simulink model "r2016bSingleARDroneCtrl"  (R2016b)
settings: Solver=FixedStepAuto  StartTime=0.0  StopTime=inf  FixedStep=sampleTime  RelTol=1e-3  EnableMultiTasking=on
values from neighbouring files (symbols this model uses):
  k_d_xy = 0.5    [start.m]
  k_d_z = 0.3    [start.m]
  k_i_xy = 0.01    [start.m]
  k_p_xy = 0.7    [start.m]
  k_p_yaw = 0.5    [start.m]
  k_p_z = 0.6    [start.m]
  limit_cmd_xy = 10    [start.m]
  waypoints1 = getWaypoints(0)    [start.m]
  waypoints2 = getWaypoints(-pi)    [start.m]
undefined symbols (not defined in the file or in its folder): Angular, Linear
libraries: robotlib x6
settings Model: Creator=exbot  LastModifiedBy=zhenglong
settings DataIOCC: LimitDataPoints=on
settings OptimizationCC: MaxStackSize=64
settings DebuggingCC: ParameterTunabilityLossMsg=error  AllowSymbolicDim=off  SFUnexpectedBacktrackingDiag=warning  SFNoUnconditionalDefaultTransitionDiag=warning  SFExecutionAtInitializationDiag=none
settings HardwareCC: ProdBitPerPointer=32  ProdBitPerSizeT=32  ProdBitPerPtrDiffT=32  ProdLargestAtomicFloat=None  ProdIntDivRoundTo=Undefined  ProdEndianess=Unspecified  ProdWordSize=32  ProdHWDeviceType=Generic->Unspecified (assume 32-bit Generic)
settings ModelReferenceCC: PropagateSignalLabelsOutOfModel=off
settings RTWCC: SystemTargetFile=ert.tlc  HardwareBoard=Robot Operating System (ROS)  TLCOptions="-aInlineSetEventsForThisBaseRateFcn=TLC_FALSE -aSuppressMultiTaskScheduler=TLC_FALSE  -aRateBasedStepFcn=0"  TemplateMakefile=ert_default_tmf  Description=Embedded Coder  Toolchain=Catkin  TargetLang=C++
settings CodeAppCC: ForceParamTrailComments=on  IgnoreCustomStorageClasses=off  OperatorAnnotations=on  SimulinkDataObjDesc=on  SFDataObjDesc=on  MATLABFcnDesc=on  InsertBlockDesc=on  MATLABSourceComments=on
settings ERTTargetCC: SupportContinuousTime=on
settings ConfigComp: CovMetricSettings=dw  CovHtmlReporting=on  CovSaveCumulativeToWorkspaceVar=on  CovSaveSingleToWorkspaceVar=on  CovExternalEMLEnable=off

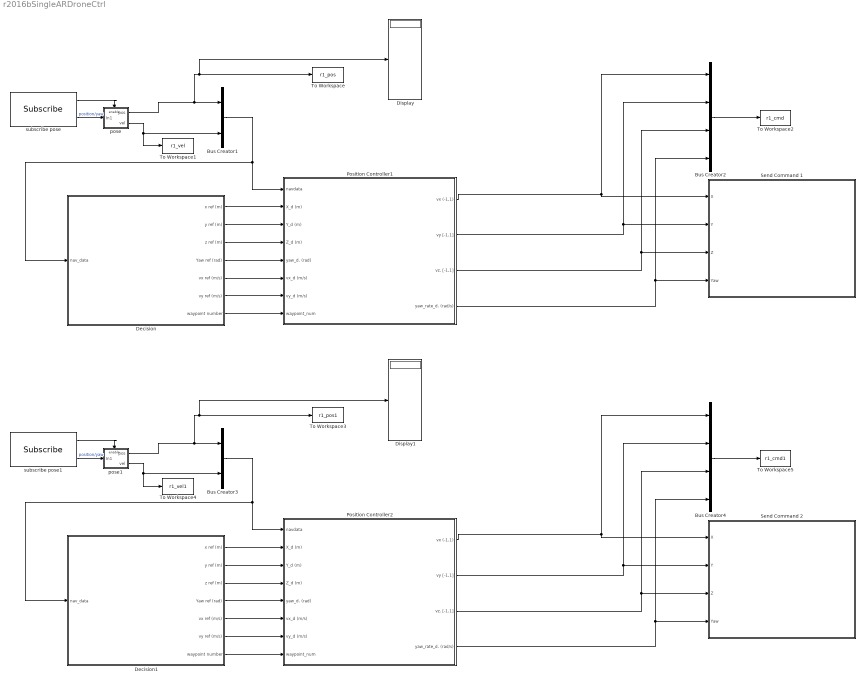
== system r2016bSingleARDroneCtrl ==
  Bus Creator1 : BusCreator  Inputs=2
  Bus Creator2 : BusCreator  Inputs=4
  Bus Creator3 : BusCreator  Inputs=2
  Bus Creator4 : BusCreator  Inputs=4
  Decision : Subsystem  AncestorBlock=ARBlocks/Guidance logic
  Decision1 : Subsystem  AncestorBlock=ARBlocks/Guidance logic
  Display : Display
  Display1 : Display
  Position Controller1 : Subsystem  AncestorBlock=ARBlocks/Baseline Controller
  Position Controller2 : Subsystem  AncestorBlock=ARBlocks/Baseline Controller
  Send Command 1 : Subsystem
  Send Command 2 : Subsystem
  To Workspace : ToWorkspace  VariableName=r1_pos  SaveFormat=Timeseries  SampleTime=-1
  To Workspace1 : ToWorkspace  VariableName=r1_vel  SaveFormat=Timeseries  SampleTime=-1
  To Workspace2 : ToWorkspace  VariableName=r1_cmd  SaveFormat=Timeseries  SampleTime=-1
  To Workspace3 : ToWorkspace  VariableName=r1_pos1  SaveFormat=Timeseries  SampleTime=-1
  To Workspace4 : ToWorkspace  VariableName=r1_vel1  SaveFormat=Timeseries  SampleTime=-1
  To Workspace5 : ToWorkspace  VariableName=r1_cmd1  SaveFormat=Timeseries  SampleTime=-1
  pose : Subsystem
  pose1 : Subsystem
  subscribe pose : robotlib/Subscribe  SourceLibraryInfo=This block requires Robotics System Toolbox  topicSource=Select from ROS network  topic=/uav1/ground_truth/state  messageType=nav_msgs/Odometry  sampleTime=-1  messageQueueLength=1
      link override SourceBlock: ROSTopic=/uav1/ground_truth/state  ROSMessageType=nav_msgs/Odometry  SLBusName=SL_Bus_SingleARDroneCtrl_nav_msgs_Odometry  ModelName=SingleARDroneCtrl  BlockId=Sub_SingleARDroneCtrl_313
  subscribe pose1 : robotlib/Subscribe  SourceLibraryInfo=This block requires Robotics System Toolbox  topicSource=Select from ROS network  topic=/uav2/ground_truth/state  messageType=nav_msgs/Odometry  sampleTime=-1  messageQueueLength=1
      link override SourceBlock: ROSTopic=/uav1/ground_truth/state  ROSMessageType=nav_msgs/Odometry  SLBusName=SL_Bus_SingleARDroneCtrl_nav_msgs_Odometry  ModelName=SingleARDroneCtrl  BlockId=Sub_SingleARDroneCtrl_313
  wires:
  Position Controller1/2(vy [-1,1]) -> Bus Creator2/2, Send Command 1/2(Y)
  Position Controller1/3(vz. [-1,1]) -> Bus Creator2/3, Send Command 1/3(Z)
  Position Controller1/4(yaw_rate_d. (rad/s)) -> Bus Creator2/4, Send Command 1/4(Yaw)
  Bus Creator2/1 -> To Workspace2/1
  subscribe pose/2 -> pose/1(In1)  "position/yaw"
  subscribe pose/1 -> pose/Enable
  pose/1(pos) -> Bus Creator1/1, Display/1, To Workspace/1
  pose/2(vel) -> Bus Creator1/2, To Workspace1/1
  Position Controller1/1(vx (-1,1)) -> Send Command 1/1(X), Bus Creator2/1
  Decision/1(x ref (m)) -> Position Controller1/2(X_d (m))
  Decision/2(y ref (m)) -> Position Controller1/3(Y_d (m))
  Decision/3(z ref (m)) -> Position Controller1/4(Z_d (m))
  Decision/4(Yaw ref (rad)) -> Position Controller1/5(yaw_d. (rad))
  Decision/5(vx ref (m/s)) -> Position Controller1/6(vx_d (m/s))
  Decision/6(vy ref (m/s)) -> Position Controller1/7(vy_d (m/s))
  Bus Creator1/1 -> Decision/1(nav_data), Position Controller1/1(navdata)
  Decision/7(waypoint number) -> Position Controller1/8(waypoint_num)
  Position Controller2/2(vy [-1,1]) -> Bus Creator4/2, Send Command 2/2(Y)
  Position Controller2/3(vz. [-1,1]) -> Bus Creator4/3, Send Command 2/3(Z)
  Position Controller2/4(yaw_rate_d. (rad/s)) -> Bus Creator4/4, Send Command 2/4(Yaw)
  Bus Creator4/1 -> To Workspace5/1
  subscribe pose1/2 -> pose1/1(In1)  "position/yaw"
  subscribe pose1/1 -> pose1/Enable
  pose1/1(pos) -> Bus Creator3/1, Display1/1, To Workspace3/1
  pose1/2(vel) -> Bus Creator3/2, To Workspace4/1
  Position Controller2/1(vx (-1,1)) -> Send Command 2/1(X), Bus Creator4/1
  Decision1/1(x ref (m)) -> Position Controller2/2(X_d (m))
  Decision1/2(y ref (m)) -> Position Controller2/3(Y_d (m))
  Decision1/3(z ref (m)) -> Position Controller2/4(Z_d (m))
  Decision1/4(Yaw ref (rad)) -> Position Controller2/5(yaw_d. (rad))
  Decision1/5(vx ref (m/s)) -> Position Controller2/6(vx_d (m/s))
  Decision1/6(vy ref (m/s)) -> Position Controller2/7(vy_d (m/s))
  Bus Creator3/1 -> Position Controller2/1(navdata), Decision1/1(nav_data)
  Decision1/7(waypoint number) -> Position Controller2/8(waypoint_num)

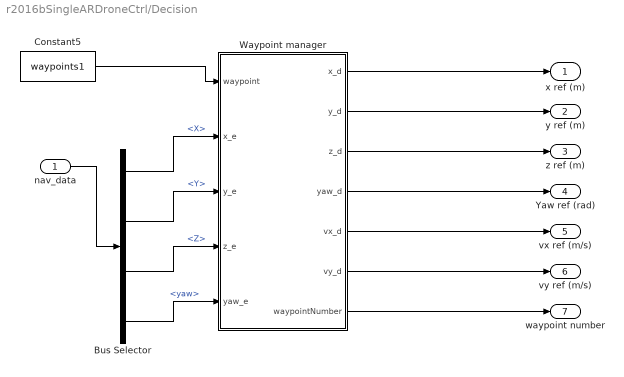
== system r2016bSingleARDroneCtrl/Decision ==
  nav_data : Inport
  Bus Selector : BusSelector  OutputSignals=signal1.X,signal1.Y,signal1.Z,signal1.yaw
  Constant5 : Constant  Value=waypoints1  VectorParams1D=off
  "Waypoint manager " : MATLAB Function  TreatAsAtomicUnit=on
  x ref (m) : Outport
  y ref (m) : Outport  Port=2
  z ref (m) : Outport  Port=3
  Yaw ref (rad) : Outport  Port=4
  vx ref (m/s) : Outport  Port=5
  vy ref (m/s) : Outport  Port=6
  waypoint number : Outport  Port=7
  wires:
  Constant5/1 -> "Waypoint manager "/1(waypoint)
  nav_data/1 -> Bus Selector/1
  "Waypoint manager "/7(waypointNumber) -> waypoint number/1
  Bus Selector/1 -> "Waypoint manager "/2(x_e)  "<X>"
  Bus Selector/2 -> "Waypoint manager "/3(y_e)  "<Y>"
  "Waypoint manager "/1(x_d) -> x ref (m)/1
  "Waypoint manager "/2(y_d) -> y ref (m)/1
  "Waypoint manager "/3(z_d) -> z ref (m)/1
  "Waypoint manager "/4(yaw_d) -> Yaw ref (rad)/1
  "Waypoint manager "/5(vx_d) -> vx ref (m/s)/1
  "Waypoint manager "/6(vy_d) -> vy ref (m/s)/1
  Bus Selector/3 -> "Waypoint manager "/4(z_e)  "<Z>"
  Bus Selector/4 -> "Waypoint manager "/5(yaw_e)  "<yaw>"

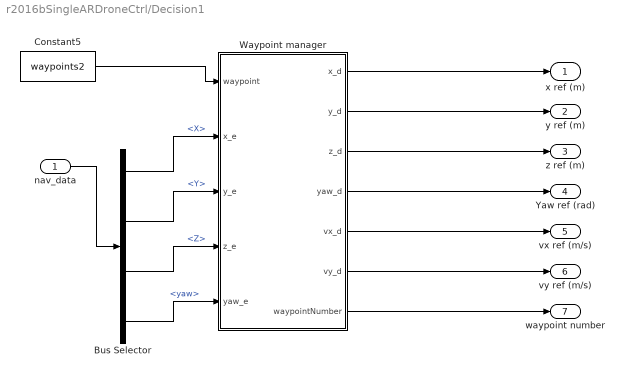
== system r2016bSingleARDroneCtrl/Decision1 ==
  nav_data : Inport
  Bus Selector : BusSelector  OutputSignals=signal1.X,signal1.Y,signal1.Z,signal1.yaw
  Constant5 : Constant  Value=waypoints2  VectorParams1D=off
  "Waypoint manager " : MATLAB Function  TreatAsAtomicUnit=on
  x ref (m) : Outport
  y ref (m) : Outport  Port=2
  z ref (m) : Outport  Port=3
  Yaw ref (rad) : Outport  Port=4
  vx ref (m/s) : Outport  Port=5
  vy ref (m/s) : Outport  Port=6
  waypoint number : Outport  Port=7
  wires:
  Constant5/1 -> "Waypoint manager "/1(waypoint)
  nav_data/1 -> Bus Selector/1
  "Waypoint manager "/7(waypointNumber) -> waypoint number/1
  Bus Selector/1 -> "Waypoint manager "/2(x_e)  "<X>"
  Bus Selector/2 -> "Waypoint manager "/3(y_e)  "<Y>"
  "Waypoint manager "/1(x_d) -> x ref (m)/1
  "Waypoint manager "/2(y_d) -> y ref (m)/1
  "Waypoint manager "/3(z_d) -> z ref (m)/1
  "Waypoint manager "/4(yaw_d) -> Yaw ref (rad)/1
  "Waypoint manager "/5(vx_d) -> vx ref (m/s)/1
  "Waypoint manager "/6(vy_d) -> vy ref (m/s)/1
  Bus Selector/3 -> "Waypoint manager "/4(z_e)  "<Z>"
  Bus Selector/4 -> "Waypoint manager "/5(yaw_e)  "<yaw>"

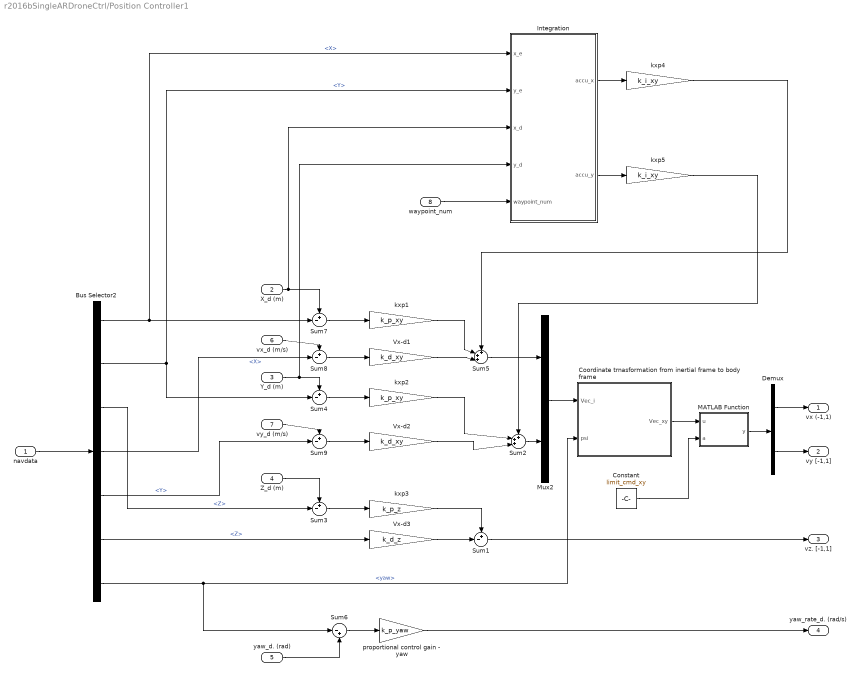
== system r2016bSingleARDroneCtrl/Position Controller1 ==
  navdata : Inport
  X_d (m) : Inport  Port=2
  Y_d (m) : Inport  Port=3
  Z_d (m) : Inport  Port=4
  yaw_d. (rad) : Inport  Port=5
  vx_d (m/s) : Inport  Port=6
  vy_d (m/s) : Inport  Port=7
  waypoint_num : Inport  Port=8
  Bus Selector2 : BusSelector  OutputSignals=signal1.X,signal1.Y,signal1.Z,signal2.X,signal2.Y,signal2.Z,signal1.yaw
  Constant : Constant  Value=limit_cmd_xy
  "Coordinate trnasformation from inertial frame to body frame " : MATLAB Function  TreatAsAtomicUnit=on
  Demux : Demux  Outputs=2
  "Integration " : MATLAB Function  TreatAsAtomicUnit=on
  MATLAB Function : MATLAB Function  TreatAsAtomicUnit=on
  Mux2 : Mux  Inputs=2
  Sum{1,3..4,7..9} (6 alike) : Sum  Inputs=+-|
  Sum2 : Sum  Inputs=+++|
  Sum5 : Sum  Inputs=+++|
  Sum6 : Sum  Inputs=|-+
  Vx-d1 : Gain  Gain=k_d_xy
  Vx-d2 : Gain  Gain=k_d_xy
  Vx-d3 : Gain  Gain=k_d_z
  kxp1 : Gain  Gain=k_p_xy
  kxp2 : Gain  Gain=k_p_xy
  kxp3 : Gain  Gain=k_p_z
  kxp4 : Gain  Gain=k_i_xy
  kxp5 : Gain  Gain=k_i_xy
  proportional control gain - yaw : Gain  Gain=k_p_yaw
  vx (-1,1) : Outport
  vy [-1,1] : Outport  Port=2
  vz. [-1,1] : Outport  Port=3
  yaw_rate_d. (rad/s) : Outport  Port=4
  wires:
  MATLAB Function/1(y) -> Demux/1
  Demux/1 -> vx (-1,1)/1
  Demux/2 -> vy [-1,1]/1
  Constant/1 -> MATLAB Function/2(a)
  Mux2/1 -> "Coordinate trnasformation from inertial frame to body frame "/1(Vec_i)
  Sum7/1 -> kxp1/1
  kxp1/1 -> Sum5/2
  Vx-d1/1 -> Sum5/3
  X_d (m)/1 -> "Integration "/3(x_d), Sum7/1
  Sum4/1 -> kxp2/1
  kxp2/1 -> Sum2/2
  Vx-d2/1 -> Sum2/3
  Y_d (m)/1 -> "Integration "/4(y_d), Sum4/1
  Sum3/1 -> kxp3/1
  kxp3/1 -> Sum1/1
  Vx-d3/1 -> Sum1/2
  Z_d (m)/1 -> Sum3/1
  Bus Selector2/1 -> "Integration "/1(x_e), Sum7/2  "<X>"
  Bus Selector2/2 -> "Integration "/2(y_e), Sum4/2  "<Y>"
  Bus Selector2/3 -> Sum3/2  "<Z>"
  Bus Selector2/6 -> Vx-d3/1  "<Z>"
  Bus Selector2/7 -> Sum6/1, "Coordinate trnasformation from inertial frame to body frame "/2(psi)  "<yaw>"
  Sum6/1 -> proportional control gain - yaw/1
  proportional control gain - yaw/1 -> yaw_rate_d. (rad/s)/1
  yaw_d. (rad)/1 -> Sum6/2
  navdata/1 -> Bus Selector2/1
  Sum5/1 -> Mux2/1
  Sum2/1 -> Mux2/2
  Sum1/1 -> vz. [-1,1]/1
  "Coordinate trnasformation from inertial frame to body frame "/1(Vec_xy) -> MATLAB Function/1(u)
  Bus Selector2/4 -> Sum8/2  "<X>"
  vx_d (m/s)/1 -> Sum8/1
  Sum8/1 -> Vx-d1/1
  Sum9/1 -> Vx-d2/1
  Bus Selector2/5 -> Sum9/2  "<Y>"
  vy_d (m/s)/1 -> Sum9/1
  waypoint_num/1 -> "Integration "/5(waypoint_num)
  "Integration "/1(accu_x) -> kxp4/1
  "Integration "/2(accu_y) -> kxp5/1
  kxp4/1 -> Sum5/1
  kxp5/1 -> Sum2/1

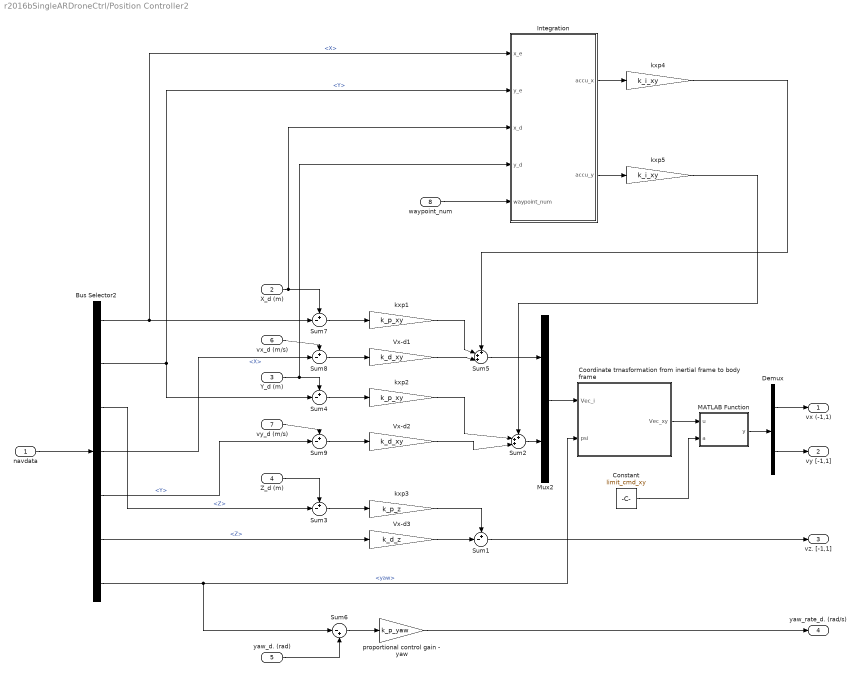
== system r2016bSingleARDroneCtrl/Position Controller2 ==
  navdata : Inport
  X_d (m) : Inport  Port=2
  Y_d (m) : Inport  Port=3
  Z_d (m) : Inport  Port=4
  yaw_d. (rad) : Inport  Port=5
  vx_d (m/s) : Inport  Port=6
  vy_d (m/s) : Inport  Port=7
  waypoint_num : Inport  Port=8
  Bus Selector2 : BusSelector  OutputSignals=signal1.X,signal1.Y,signal1.Z,signal2.X,signal2.Y,signal2.Z,signal1.yaw
  Constant : Constant  Value=limit_cmd_xy
  "Coordinate trnasformation from inertial frame to body frame " : MATLAB Function  TreatAsAtomicUnit=on
  Demux : Demux  Outputs=2
  "Integration " : MATLAB Function  TreatAsAtomicUnit=on
  MATLAB Function : MATLAB Function  TreatAsAtomicUnit=on
  Mux2 : Mux  Inputs=2
  Sum{1,3..4,7..9} (6 alike) : Sum  Inputs=+-|
  Sum2 : Sum  Inputs=+++|
  Sum5 : Sum  Inputs=+++|
  Sum6 : Sum  Inputs=|-+
  Vx-d1 : Gain  Gain=k_d_xy
  Vx-d2 : Gain  Gain=k_d_xy
  Vx-d3 : Gain  Gain=k_d_z
  kxp1 : Gain  Gain=k_p_xy
  kxp2 : Gain  Gain=k_p_xy
  kxp3 : Gain  Gain=k_p_z
  kxp4 : Gain  Gain=k_i_xy
  kxp5 : Gain  Gain=k_i_xy
  proportional control gain - yaw : Gain  Gain=k_p_yaw
  vx (-1,1) : Outport
  vy [-1,1] : Outport  Port=2
  vz. [-1,1] : Outport  Port=3
  yaw_rate_d. (rad/s) : Outport  Port=4
  wires:
  MATLAB Function/1(y) -> Demux/1
  Demux/1 -> vx (-1,1)/1
  Demux/2 -> vy [-1,1]/1
  Constant/1 -> MATLAB Function/2(a)
  Mux2/1 -> "Coordinate trnasformation from inertial frame to body frame "/1(Vec_i)
  Sum7/1 -> kxp1/1
  kxp1/1 -> Sum5/2
  Vx-d1/1 -> Sum5/3
  X_d (m)/1 -> "Integration "/3(x_d), Sum7/1
  Sum4/1 -> kxp2/1
  kxp2/1 -> Sum2/2
  Vx-d2/1 -> Sum2/3
  Y_d (m)/1 -> "Integration "/4(y_d), Sum4/1
  Sum3/1 -> kxp3/1
  kxp3/1 -> Sum1/1
  Vx-d3/1 -> Sum1/2
  Z_d (m)/1 -> Sum3/1
  Bus Selector2/1 -> "Integration "/1(x_e), Sum7/2  "<X>"
  Bus Selector2/2 -> "Integration "/2(y_e), Sum4/2  "<Y>"
  Bus Selector2/3 -> Sum3/2  "<Z>"
  Bus Selector2/6 -> Vx-d3/1  "<Z>"
  Bus Selector2/7 -> Sum6/1, "Coordinate trnasformation from inertial frame to body frame "/2(psi)  "<yaw>"
  Sum6/1 -> proportional control gain - yaw/1
  proportional control gain - yaw/1 -> yaw_rate_d. (rad/s)/1
  yaw_d. (rad)/1 -> Sum6/2
  navdata/1 -> Bus Selector2/1
  Sum5/1 -> Mux2/1
  Sum2/1 -> Mux2/2
  Sum1/1 -> vz. [-1,1]/1
  "Coordinate trnasformation from inertial frame to body frame "/1(Vec_xy) -> MATLAB Function/1(u)
  Bus Selector2/4 -> Sum8/2  "<X>"
  vx_d (m/s)/1 -> Sum8/1
  Sum8/1 -> Vx-d1/1
  Sum9/1 -> Vx-d2/1
  Bus Selector2/5 -> Sum9/2  "<Y>"
  vy_d (m/s)/1 -> Sum9/1
  waypoint_num/1 -> "Integration "/5(waypoint_num)
  "Integration "/1(accu_x) -> kxp4/1
  "Integration "/2(accu_y) -> kxp5/1
  kxp4/1 -> Sum5/1
  kxp5/1 -> Sum2/1

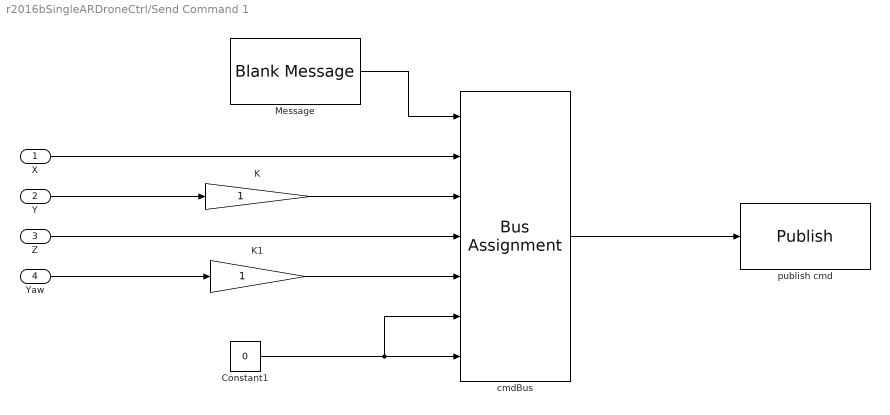
== system r2016bSingleARDroneCtrl/Send Command 1 ==
  X : Inport
  Y : Inport  Port=2
  Z : Inport  Port=3
  Yaw : Inport  Port=4
  " Message" : robotlib/Blank Message  SourceLibraryInfo=This block requires Robotics System Toolbox  messageType=geometry_msgs/Twist  SampleTime=inf
  Constant1 : Constant  Value=0
  K : Gain
  K1 : Gain
  cmdBus : BusAssignment  AssignedSignals=Linear.X,Linear.Y,Linear.Z,Angular.Z,Angular.X,Angular.Y
  publish cmd : robotlib/Publish  SourceLibraryInfo=This block requires Robotics System Toolbox  topicSource=Select from ROS network  topic=/uav1/cmd_vel  messageType=geometry_msgs/Twist  messageQueueLength=1
  wires:
  cmdBus/1 -> publish cmd/1
  Constant1/1 -> cmdBus/6, cmdBus/7
  K/1 -> cmdBus/3
  K1/1 -> cmdBus/5
  " Message"/1 -> cmdBus/1
  X/1 -> cmdBus/2
  Y/1 -> K/1
  Z/1 -> cmdBus/4
  Yaw/1 -> K1/1

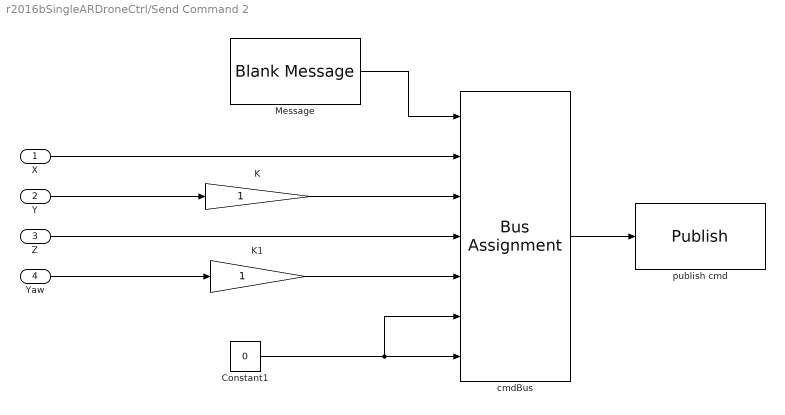
== system r2016bSingleARDroneCtrl/Send Command 2 ==
  X : Inport
  Y : Inport  Port=2
  Z : Inport  Port=3
  Yaw : Inport  Port=4
  " Message" : robotlib/Blank Message  SourceLibraryInfo=This block requires Robotics System Toolbox  messageType=geometry_msgs/Twist  SampleTime=inf
  Constant1 : Constant  Value=0
  K : Gain
  K1 : Gain
  cmdBus : BusAssignment  AssignedSignals=Linear.X,Linear.Y,Linear.Z,Angular.Z,Angular.X,Angular.Y
  publish cmd : robotlib/Publish  SourceLibraryInfo=This block requires Robotics System Toolbox  topicSource=Select from ROS network  topic=/uav2/cmd_vel  messageType=geometry_msgs/Twist  messageQueueLength=1
  wires:
  cmdBus/1 -> publish cmd/1
  Constant1/1 -> cmdBus/6, cmdBus/7
  K/1 -> cmdBus/3
  K1/1 -> cmdBus/5
  " Message"/1 -> cmdBus/1
  X/1 -> cmdBus/2
  Y/1 -> K/1
  Z/1 -> cmdBus/4
  Yaw/1 -> K1/1

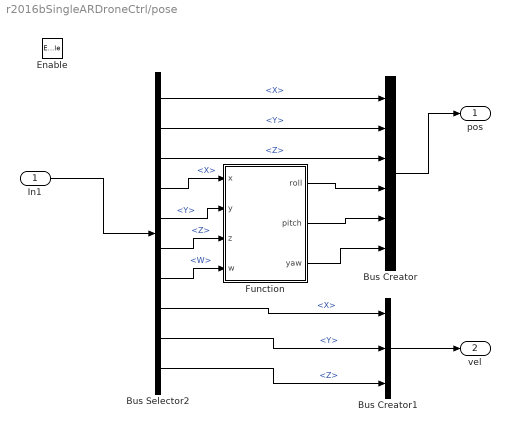
== system r2016bSingleARDroneCtrl/pose ==
  In1 : Inport
  Enable : EnablePort
  " Function" : MATLAB Function  TreatAsAtomicUnit=on
  Bus Creator : BusCreator  Inputs=6
  Bus Creator1 : BusCreator  Inputs=3
  Bus Selector2 : BusSelector  OutputSignals=Pose.Pose.Position.X,Pose.Pose.Position.Y,Pose.Pose.Position.Z,Pose.Pose.Orientation.X,Pose.Pose.Orientation.Y,Pose.Pose.Orientation.Z,Pose.Pose.Orientation.W,Twist.Twist.Linear.X,Twist.Twist.Linear.Y,Twist.Twist.Linear.Z
  pos : Outport
  vel : Outport  Port=2
  wires:
  Bus Creator/1 -> pos/1
  In1/1 -> Bus Selector2/1
  " Function"/1(roll) -> Bus Creator/4
  Bus Selector2/4 -> " Function"/1(x)  "<X>"
  Bus Selector2/5 -> " Function"/2(y)  "<Y>"
  Bus Selector2/6 -> " Function"/3(z)  "<Z>"
  Bus Selector2/7 -> " Function"/4(w)  "<W>"
  Bus Selector2/1 -> Bus Creator/1  "<X>"
  Bus Selector2/2 -> Bus Creator/2  "<Y>"
  Bus Selector2/3 -> Bus Creator/3  "<Z>"
  " Function"/2(pitch) -> Bus Creator/5
  " Function"/3(yaw) -> Bus Creator/6
  Bus Creator1/1 -> vel/1
  Bus Selector2/8 -> Bus Creator1/1  "<X>"
  Bus Selector2/9 -> Bus Creator1/2  "<Y>"
  Bus Selector2/10 -> Bus Creator1/3  "<Z>"

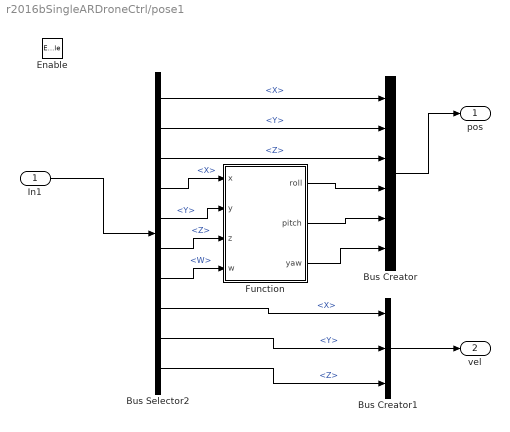
== system r2016bSingleARDroneCtrl/pose1 ==
  In1 : Inport
  Enable : EnablePort
  " Function" : MATLAB Function  TreatAsAtomicUnit=on
  Bus Creator : BusCreator  Inputs=6
  Bus Creator1 : BusCreator  Inputs=3
  Bus Selector2 : BusSelector  OutputSignals=Pose.Pose.Position.X,Pose.Pose.Position.Y,Pose.Pose.Position.Z,Pose.Pose.Orientation.X,Pose.Pose.Orientation.Y,Pose.Pose.Orientation.Z,Pose.Pose.Orientation.W,Twist.Twist.Linear.X,Twist.Twist.Linear.Y,Twist.Twist.Linear.Z
  pos : Outport
  vel : Outport  Port=2
  wires:
  Bus Creator/1 -> pos/1
  In1/1 -> Bus Selector2/1
  " Function"/1(roll) -> Bus Creator/4
  Bus Selector2/4 -> " Function"/1(x)  "<X>"
  Bus Selector2/5 -> " Function"/2(y)  "<Y>"
  Bus Selector2/6 -> " Function"/3(z)  "<Z>"
  Bus Selector2/7 -> " Function"/4(w)  "<W>"
  Bus Selector2/1 -> Bus Creator/1  "<X>"
  Bus Selector2/2 -> Bus Creator/2  "<Y>"
  Bus Selector2/3 -> Bus Creator/3  "<Z>"
  " Function"/2(pitch) -> Bus Creator/5
  " Function"/3(yaw) -> Bus Creator/6
  Bus Creator1/1 -> vel/1
  Bus Selector2/8 -> Bus Creator1/1  "<X>"
  Bus Selector2/9 -> Bus Creator1/2  "<Y>"
  Bus Selector2/10 -> Bus Creator1/3  "<Z>"

== matlab function r2016bSingleARDroneCtrl/Decision1/Waypoint manager  ==
  data: x_d output; y_d output; waypoint input; x_e input; y_e input; z_e input; yaw_e input; z_d output; yaw_d output; vx_d output; vy_d output; waypointNumber output
function [x_d, y_d,  z_d, yaw_d, vx_d,vy_d ,waypointNumber] = fcn(waypoint, x_e,y_e,z_e,yaw_e)
%#codegen
% Waypoint matrix contains final position, orientatoin, and waiting time.
% Number of waypoints
nPoints = size(waypoint, 2) ;
% Persitent variable used to keep trak of next waypoint
persistent wpointer;
% Init. persistent variables
if isempty(wpointer)
    wpointer = 1;
end
% A waypoint is reached if the distance between the desired waypoint and 
% the vehicle is less than 0.2 m in the XY plane, less than 0.2 m in height, 
if ( sqrt((x_e- waypoint(2, wpointer))^2+(y_e- waypoint(3, wpointer))^2 )< 0.5 && ...
        norm(z_e - waypoint(4, wpointer)) < 0.2  && ...
        norm(yaw_e - waypoint(5, wpointer) )< 10*pi/180 &&...
        wpointer ~= nPoints)
        wpointer = wpointer+ 1;
end


%% Outputs:
x_d = waypoint(2, wpointer) ;
y_d = waypoint(3, wpointer) ;
z_d = waypoint(4, wpointer)  ;
yaw_d = waypoint(5, wpointer) ;
vx_d = waypoint(6,wpointer);
vy_d = waypoint(7,wpointer);
waypointNumber = wpointer ;

== matlab function r2016bSingleARDroneCtrl/Position Controller2/Coordinate trnasformation from inertial frame to body frame  ==
  data: Vec_i input; Vec_xy output; psi input
function Vec_xy  = fcn(Vec_i , psi)
%#codegen
T = [cos(psi) sin(psi) ; -sin(psi) cos(psi)] ; 
Vec_xy = T*Vec_i(1:2,1);

== matlab function r2016bSingleARDroneCtrl/Position Controller2/Integration  ==
  data: x_e input; y_e input; accu_x output; accu_y output; x_d input; y_d input; waypoint_num input
function [accu_x, accu_y] = integration(x_e,y_e,x_d, y_d,waypoint_num)

persistent last_waypoint;
persistent sum_x;
persistent sum_y;
% Init. persistent variables

if isempty(last_waypoint)
    last_waypoint = 0;
end

if isempty(sum_x)
    sum_x = 0;
end
if isempty(sum_y)
    sum_y = 0;
end

if waypoint_num>last_waypoint
    sum_x = 0;
    sum_y = 0;
    last_waypoint = last_waypoint +1;
elseif last_waypoint==waypoint_num
    sum_x =sum_x +(x_d-x_e);
    sum_y =sum_y +(y_d-y_e);
end

%% Outputs:
accu_x = sum_x;
accu_y = sum_y;

== matlab function r2016bSingleARDroneCtrl/pose/ Function ==
  data: x input; roll output; y input; z input; w input; pitch output; yaw output
function [roll, pitch, yaw] = quat2rpy(x, y, z, w)
    t0 = -2.0 * (y * y + z * z) + 1.0;
    t1 = +2.0 * (x * y + w * z);
    t2 = -2.0 * (x * z - w * y);
    t3 = +2.0 * (y * z + w * x);
    t4 = -2.0 * (x * x + y * y) + 1.0;

    roll = -asin(t2);
    pitch = -atan2(t3, t4);
    yaw= -atan2(t1, t0);

== matlab function r2016bSingleARDroneCtrl/Position Controller1/MATLAB Function ==
  data: u input; y output; a input
function y = fcn(u,a)
    temp = norm(u,Inf);
    if  temp<=a
        y = u;
    else
        y= a*u/temp;
    end
end

== matlab function r2016bSingleARDroneCtrl/Position Controller2/MATLAB Function ==
  data: u input; y output; a input
function y = fcn(u,a)
    temp = norm(u,Inf);
    if  temp<=a
        y = u;
    else
        y= a*u/temp;
    end
end

== matlab function r2016bSingleARDroneCtrl/Position Controller1/Integration  ==
  data: x_e input; y_e input; accu_x output; accu_y output; x_d input; y_d input; waypoint_num input
function [accu_x, accu_y] = integration(x_e,y_e,x_d, y_d,waypoint_num)

persistent last_waypoint;
persistent sum_x;
persistent sum_y;
% Init. persistent variables

if isempty(last_waypoint)
    last_waypoint = 0;
end

if isempty(sum_x)
    sum_x = 0;
end
if isempty(sum_y)
    sum_y = 0;
end

if waypoint_num>last_waypoint
    sum_x = 0;
    sum_y = 0;
    last_waypoint = last_waypoint +1;
elseif last_waypoint==waypoint_num
    sum_x =sum_x +(x_d-x_e);
    sum_y =sum_y +(y_d-y_e);
end

%% Outputs:
accu_x = sum_x;
accu_y = sum_y;

== matlab function r2016bSingleARDroneCtrl/pose1/ Function ==
  data: x input; roll output; y input; z input; w input; pitch output; yaw output
function [roll, pitch, yaw] = quat2rpy(x, y, z, w)
    t0 = -2.0 * (y * y + z * z) + 1.0;
    t1 = +2.0 * (x * y + w * z);
    t2 = -2.0 * (x * z - w * y);
    t3 = +2.0 * (y * z + w * x);
    t4 = -2.0 * (x * x + y * y) + 1.0;

    roll = -asin(t2);
    pitch = -atan2(t3, t4);
    yaw= -atan2(t1, t0);

== matlab function r2016bSingleARDroneCtrl/Decision/Waypoint manager  ==
  data: x_d output; y_d output; waypoint input; x_e input; y_e input; z_e input; yaw_e input; z_d output; yaw_d output; vx_d output; vy_d output; waypointNumber output
function [x_d, y_d,  z_d, yaw_d, vx_d,vy_d ,waypointNumber] = fcn(waypoint, x_e,y_e,z_e,yaw_e)
%#codegen
% Waypoint matrix contains final position, orientatoin, and waiting time.
% Number of waypoints
nPoints = size(waypoint, 2) ;
% Persitent variable used to keep trak of next waypoint
persistent wpointer;
% Init. persistent variables
if isempty(wpointer)
    wpointer = 1;
end
% A waypoint is reached if the distance between the desired waypoint and 
% the vehicle is less than 0.2 m in the XY plane, less than 0.2 m in height, 
if ( sqrt((x_e- waypoint(2, wpointer))^2+(y_e- waypoint(3, wpointer))^2 )< 0.5 && ...
        norm(z_e - waypoint(4, wpointer)) < 0.2  && ...
        norm(yaw_e - waypoint(5, wpointer) )< 10*pi/180 &&...
        wpointer ~= nPoints)
        wpointer = wpointer+ 1;
end


%% Outputs:
x_d = waypoint(2, wpointer) ;
y_d = waypoint(3, wpointer) ;
z_d = waypoint(4, wpointer)  ;
yaw_d = waypoint(5, wpointer) ;
vx_d = waypoint(6,wpointer);
vy_d = waypoint(7,wpointer);
waypointNumber = wpointer ;

== matlab function r2016bSingleARDroneCtrl/Position Controller1/Coordinate trnasformation from inertial frame to body frame  ==
  data: Vec_i input; Vec_xy output; psi input
function Vec_xy  = fcn(Vec_i , psi)
%#codegen
T = [cos(psi) sin(psi) ; -sin(psi) cos(psi)] ; 
Vec_xy = T*Vec_i(1:2,1);
